simulink library "ddm"  (R2021b)
settings: Solver=VariableStepAuto  StartTime=0.0  StopTime=10.0  RelTol=1e-3
undefined symbols (not defined in the file or in its folder): ENUM_ADASACCSTA_ERROR, ENUM_ADASACCSTA_OFF, ENUM_ADASACCSTA_STANDBY, ENUM_ADASISASTA_OFF, ENUM_ALLOWMOV_ALLOWREADY, ENUM_APS, ENUM_BRKSTA_ERROR, ENUM_BRKSTA_OFF, ENUM_BRKSTA_ON, ENUM_CHGPREACTERRSTA_OBCPRE, ENUM_DCDCFAULTSTA_ANYFAULTLV1, ENUM_DCDCFAULTSTA_ANYFAULTLV2, ENUM_DRIVETRAIN_AWD, ENUM_DRIVETRAIN_FWD, ENUM_DRIVETRAIN_RWD, ENUM_DRSEATSTA_INVALID, ENUM_EDUDRTSTA_NORMAL, ENUM_EPBSTA_APPLIED, ENUM_EPBSTA_RELEASED, ENUM_HVBATTREADYPRE_READY, ENUM_MCUWARN_LV0, ENUM_MCUWARN_LV1, ENUM_MCUWARN_LV2, ENUM_MCUWARN_LV3, ENUM_MCUWARN_NOERROR, ENUM_OBCFAULTSTA_ANYFAULT, ENUM_PAS_R2F2, ENUM_PDFAULT_BATTPDFAIL, ENUM_PDFAULT_DCDCDISABLE, ENUM_PDFAULT_MCUDISABLE, ENUM_PDFAULT_MCUDISCHRG, ENUM_POWERSTA_OFF, ENUM_POWERSTA_ON, ENUM_POWERSTA_READY, ENUM_POWERSTA_STANDBY, ENUM_PRESSINDI_LOW, ENUM_PUFAULT_BATTUPFAIL, ENUM_PUFAULT_DCDCENABLEFAIL, ENUM_PUFAULT_PRECHRGCHKFAIL, ENUM_PUFAULT_SAFETYCHKFAIL, ENUM_PUSTATE_COMPLETED, ENUM_PWRSTASW_OFF, ENUM_PWRSTASW_OFFA, ENUM_PWRSTASW_OFFCHVCHRG, ENUM_PWRSTASW_OFFCLVCHRG, ENUM_PWRSTASW_ON, ENUM_PWRSTASW_ONHVCHRG, ENUM_PWRSTASW_READY, ENUM_PWRSTASW_STANDBY, ENUM_RANGESTA_12IN, ENUM_RANGESTA_12OUT, ENUM_SHIFTCOMMAND_D, ENUM_SHIFTCOMMAND_N, ENUM_SHIFTCOMMAND_P, ENUM_SHIFTCOMMAND_R, ENUM_ZONEMALFUNLV_1ST, ENUM_ZONEMALFUNLV_2ND, ENUM_ZONEMALFUNLV_3RD, ENUM_ZONEMALFUNLV_4TH, ENUM_ZONESPDCTRLMODE_ACC ... (+832)
libraries: hcu_lib x738, $bdroot x26, simulink x7
(part 16 of 25)

== system ddm/DDM/DDM/PMM/Fault level/Fault level 4 subsystem error ==
  note: Fail Safe Operation During Failure Detection
  note: Test Detection Criteria
  note: Diagnostics and Fault Handling
  note: Release Condition After Failure Decision
  note: Release Condition During Failure Detection
  note: Test Pass Criteria
  note: Fail Safe Operation After Failure Decision
  task_time_s : Inport
  VPMM_PowerSta_enum : Inport  Port=2
  VPMM_PwrStaSW_enum : Inport  Port=3
  VDDM_C3BMS6LCCFS_flg : Inport  Port=4
  VINP_BMSWarn7_flg : Inport  Port=5
  VINP_BMSWarn8_flg : Inport  Port=6
  DTC_clear_request : Inport  Port=7
  No_CAN3_BUS_OFF : Inport  Port=8
  Constant10 : Constant  Value=KDDM_Lv4ErrDetSW_flg
  Constant11 : Constant  Value=KDDM_Lv4ErrPassSW_flg
  Constant15 : Constant  Value=KDDM_Lv4ErrCFSSW_flg
  Constant16 : Constant  Value=TRUE
  Constant18 : Constant  Value=KDDM_Lv4ErrPassTO_s
  Constant19 : Constant  Value=ENUM_POWERSTA_OFF
  Constant{2,21,25,27} (4 alike) : Constant  Value=FALSE
  Constant20 : Constant  Value=KDDM_Lv4ErrDFSSW_flg
  Constant22 : Constant  Value=ENUM_PWRSTASW_OFF
  Constant23 : Constant  Value=TRUE
  Constant24 : Constant  Value=TRUE
  Constant26 : Constant  Value=ENUM_PWRSTASW_OFF
  Constant3 : Constant  Value=KDDM_Lv4ErrDetTO_s
  Constant4 : Constant  Value=KDDM_Lv4ErrPassTO_s
  Constant40 : Constant  Value=KDDM_Lv4ErrDTC_cnt
  Constant5 : Constant  Value=KDDM_Lv4ErrDTC_cnt
  DTC_Couter : hcu_lib/Basic_Blocks/DTC_Couter
  DTC_Info : hcu_lib/Basic_Blocks/DTC_Info
  Data Type Conversion1 : DataTypeConversion  OutDataTypeStr=uint8
  Equal : RelationalOperator  Operator=~=  OutDataTypeStr=boolean  RndMeth=Simplest
  Equal2 : RelationalOperator  Operator=~=  OutDataTypeStr=boolean  RndMeth=Simplest
  Equal3 : RelationalOperator  OutDataTypeStr=boolean  RndMeth=Simplest
  Equal4 : RelationalOperator  Operator===  OutDataTypeStr=boolean  RndMeth=Simplest
  Goto24 : Goto  Commented=on  GotoTag=VDDM_EDriveSysErrVCUErr_flg
  Logical Operator1 : Logic  Operator=NOT  AllPortsSameDT=off  OutDataTypeStr=boolean
  Logical Operator{3,5,8,11} (4 alike) : Logic  Operator=OR  AllPortsSameDT=off  OutDataTypeStr=boolean
  Logical Operator{12,15,18..19} (4 alike) : Logic  AllPortsSameDT=off  OutDataTypeStr=boolean
  Logical Operator2 : Logic  Inputs=3  AllPortsSameDT=off  OutDataTypeStr=boolean
  Logical Operator4 : Logic  Operator=NOT  AllPortsSameDT=off  OutDataTypeStr=boolean
  Logical Operator6 : Logic  Operator=NOT  AllPortsSameDT=off  OutDataTypeStr=boolean
  Logical Operator7 : Logic  Inputs=3  AllPortsSameDT=off  OutDataTypeStr=boolean
  Relay : Relay  OnSwitchValue=ONE_INT  OffSwitchValue=ZERO_INT
  SR_Latch1 : Subsystem  mask(SR_Latch){}
      mask help: SR latch function.
  SR_Latch3 : hcu_lib/Basic_Blocks/SR_Latch
  SR_Latch4 : hcu_lib/Basic_Blocks/SR_Latch
  Switch{,2,4..6} (5 alike) : Switch  Criteria=u2 ~= 0
  Test Detection Criteria : hcu_lib/Basic_Blocks/Test Detection Criteria
  Timer1 : hcu_lib/Basic_Blocks/Timer
  VDDM_Lv4ErrDTC_raw32 : Outport
  wires:
  VINP_BMSWarn8_flg/1 -> [VINP_BMSWarn8_flg]
  VPMM_PowerSta_enum/1 -> [VPMM_PowerSta_enum]
  VPMM_PwrStaSW_enum/1 -> [VPMM_PwrStaSW_enum]
  task_time_s/1 -> [task_time_s]
  VINP_BMSWarn7_flg/1 -> [VINP_BMSWarn7_flg]
  VDDM_C3BMS6LCCFS_flg/1 -> [VDDM_C3BMS6LCCFS_flg]
  [VDDM_Lv4ErrCFSRls_flg] -> Logical Operator3/2
  Constant10/1 -> Logical Operator19/2
  SR_Latch1/1(latched) -> [VDDM_Lv4ErrPass_flg]  "VDDM_Lv4ErrPass_flg"
  [VINP_BMSWarn7_flg] -> Logical Operator11/1
  Constant5/1 -> DTC_Couter/3
  Constant11/1 -> Logical Operator15/2
  Constant20/1 -> Logical Operator12/1
  [No_CAN3_BUS_OFF] -> Logical Operator2/1
  Logical Operator6/1 -> Timer1/1
  [task_time_s] -> Test Detection Criteria/2
  [VDDM_Lv4ErrCFS_flg] -> Switch/2
  [VDDM_C3BMS6LCCFS_flg] -> Logical Operator1/1
  DTC_Couter/2 -> Data Type Conversion1/1
  Switch/1 -> Goto24/1
  Equal3/1 -> SR_Latch1/1(set)
  Constant40/1 -> Test Detection Criteria/3
  Equal4/1 -> Logical Operator8/1
  [DTC_clear_request] -> Logical Operator8/2
  Timer1/1 -> Equal3/1
  Constant26/1 -> Equal/2
  Constant18/1 -> Equal3/2
  Logical Operator18/1 -> [VDDM_Lv4ErrCFS_flg]
  Data Type Conversion1/1 -> [VDDM_Lv4ErrDTC_cnt]  "VDDM_Lv4ErrDTC_cnt"
  Logical Operator1/1 -> Logical Operator2/3
  Constant24/1 -> Switch4/1
  SR_Latch3/1 -> Logical Operator12/2
  Logical Operator19/1 -> DTC_Couter/1
  Logical Operator15/1 -> DTC_Couter/2
  Logical Operator2/1 -> Switch5/2
  Logical Operator3/1 -> Logical Operator15/1
  Switch2/1 -> Logical Operator6/1, Timer1/2
  DTC_Couter/1 -> SR_Latch4/1
  Logical Operator8/1 -> Switch4/2
  Logical Operator12/1 -> [VDDM_Lv4ErrDFS_flg]
  Constant16/1 -> Switch/1
  Switch4/1 -> [VDDM_Lv4ErrCFSRls_flg]
  Constant15/1 -> Logical Operator18/2
  [VDDM_Lv4ErrCFSRls_flg] -> SR_Latch4/2
  [VDDM_Lv4ErrPass_flg] -> Logical Operator3/1
  Relay/1 -> SR_Latch3/1
  Constant27/1 -> Switch5/3
  Equal/1 -> Logical Operator2/2
  Constant21/1 -> Switch/3
  Test Detection Criteria/1 -> [VDDM_Lv4ErrDet_flg]  "VDDM_Lv4ErrDet_flg"
  Logical Operator11/1 -> Switch5/1
  Constant25/1 -> Switch4/3
  Constant19/1 -> Equal4/2
  [VDDM_Lv4ErrDTC_cnt] -> Relay/1
  Constant4/1 -> Timer1/4
  SR_Latch4/1 -> Logical Operator18/1
  [VDDM_Lv4ErrDet_flg] -> Logical Operator19/1
  [VINP_BMSWarn8_flg] -> Logical Operator11/2
  [VINP_BMSWarn8_flg] -> Logical Operator5/2
  Logical Operator5/1 -> Switch2/1
  Equal2/1 -> Logical Operator7/2
  Constant23/1 -> Switch2/3
  Constant22/1 -> Equal2/2
  Logical Operator7/1 -> Switch2/2
  Logical Operator4/1 -> Logical Operator7/3
  [VPMM_PwrStaSW_enum] -> Equal2/1
  [VDDM_C3BMS6LCCFS_flg] -> Logical Operator4/1
  [No_CAN3_BUS_OFF] -> Logical Operator7/1
  [VINP_BMSWarn7_flg] -> Logical Operator5/1
  [VPMM_PowerSta_enum] -> Equal4/1
  [VPMM_PwrStaSW_enum] -> Equal/1
  DTC_clear_request/1 -> [DTC_clear_request]
  No_CAN3_BUS_OFF/1 -> [No_CAN3_BUS_OFF]
  [task_time_s] -> Timer1/3
  DTC_Info/1 -> VDDM_Lv4ErrDTC_raw32/1  "VDDM_Lv4ErrDTC_raw32"
  [VDDM_Lv4ErrPass_flg] -> DTC_Info/2
  [VDDM_Lv4ErrCFS_flg] -> DTC_Info/3
  [VDDM_Lv4ErrCFS_flg] -> SR_Latch3/2
  [VDDM_Lv4ErrDet_flg] -> DTC_Info/1
  Constant3/1 -> Test Detection Criteria/4
  [DTC_clear_request] -> DTC_Info/4
  [DTC_clear_request] -> Switch6/2
  Switch6/1 -> Test Detection Criteria/1
  Switch5/1 -> [VDDM_xxx_flg], Switch6/3
  Constant2/1 -> Switch6/1
  [VDDM_xxx_flg] -> SR_Latch1/2(reset)

== system ddm/DDM/DDM/PMM/Key authentication failed/SR_Latch1 ==
  set : Inport
  reset : Inport  Port=2
  Logical Operator : Logic  AllPortsSameDT=off  OutDataTypeStr=boolean
  Logical Operator1 : Logic  Operator=NOT  AllPortsSameDT=off  OutDataTypeStr=boolean
  Switch1 : Switch  Criteria=u2 ~= 0  Threshold=0.5
      settings: AttributesFormatString=<Criteria=%<Criteria>>
  Switch2 : Switch  Criteria=u2 ~= 0  Threshold=0.5
      settings: AttributesFormatString=<Criteria=%<Criteria>>
  Unit Delay : UnitDelay  SampleTime=-1  HasFrameUpgradeWarning=on
  latched : Outport
  wires:
  Switch1/1 -> Unit Delay/1, latched/1
  set/1 -> Switch1/1, Logical Operator/1
  reset/1 -> Switch2/2, Logical Operator1/1
  Unit Delay/1 -> Switch2/3
  Switch2/1 -> Switch1/3
  Logical Operator/1 -> Switch1/2
  Logical Operator1/1 -> Logical Operator/2, Switch2/1

== system ddm/DDM/DDM/PMM/LV/Initial LV battery voltage too low ==
  note: Test Detection Criteria
  note: Test Pass Criteria
  note: Fail Safe After Decision
  note: Fail Safe During Detection
  note: Release Condition During Detection
  note: Release Condition After Decision
  note: Diagnostics and Fault Handling
  task_time_s : Inport
  VPMM_PowerSta_enum : Inport  Port=2
  VPMM_PwrStaSW_enum : Inport  Port=3
  VINP_LVBattDet12V_V : Inport  Port=4
  VINP_CANMsgValidBMS2_flg : Inport  Port=5
  DTC_clear_request : Inport  Port=6
  Constant1 : Constant  Value=TRUE
  Constant10 : Constant  Value=ENUM_POWERSTA_OFF
  Constant11 : Constant  Value=KDDM_IniLVLoPassSW_flg
  Constant15 : Constant  Value=KDDM_IniLVLoCFSSW_flg
  Constant16 : Constant  Value=TRUE
  Constant18 : Constant  Value=KDDM_IniLVLoPassTO_s
  Constant19 : Constant  Value=KDDM_IniLVLoPassTO_s
  Constant2 : Constant  Value=ENUM_PWRSTASW_STANDBY
  Constant20 : Constant  Value=KDDM_IniLVLoDFSSW_flg
  Constant{4,8,21,25} (4 alike) : Constant  Value=FALSE
  Constant24 : Constant  Value=TRUE
  Constant3 : Constant  Value=ENUM_PWRSTASW_OFF
  Constant40 : Constant  Value=KDDM_IniLVLoDTC_cnt
  Constant41 : Constant  Value=KDDM_IniLVLoDetTO_s
  Constant46 : Constant  Value=KDDM_IniLVLoDetSW_flg
  Constant48 : Constant  Value=KDDM_IniLVLoDTC_cnt
  Constant5 : Constant  Value=ENUM_PWRSTASW_STANDBY
  Constant6 : Constant  Value=KDDM_IniLVLoThd_mv
  Constant7 : Constant  Value=ENUM_PWRSTASW_OFF
  Constant9 : Constant  Value=KDDM_IniLVLoThd_mv
  DTC_Couter : hcu_lib/Basic_Blocks/DTC_Couter
  DTC_Info : hcu_lib/Basic_Blocks/DTC_Info
  Data Type Conversion1 : DataTypeConversion  OutDataTypeStr=uint8
  Equal{,1..2,4,6} (5 alike) : RelationalOperator  Operator===  OutDataTypeStr=boolean  RndMeth=Simplest
  Equal3 : RelationalOperator  OutDataTypeStr=boolean  RndMeth=Simplest
  Equal5 : RelationalOperator  Operator=<=  OutDataTypeStr=boolean  RndMeth=Simplest
  Equal7 : RelationalOperator  Operator=<=  OutDataTypeStr=boolean  RndMeth=Simplest
  Gain1 : Gain  Gain=1000
  Gain2 : Gain  Gain=1000
  Goto6 : Goto  Commented=on  GotoTag=VDDM_EDriveSysErrVCUErr_flg
  Logical Operator{1..2,12,15,18..19} (6 alike) : Logic  AllPortsSameDT=off  OutDataTypeStr=boolean
  Logical Operator3 : Logic  Operator=OR  AllPortsSameDT=off  OutDataTypeStr=boolean
  Logical Operator6 : Logic  Operator=NOT  AllPortsSameDT=off  OutDataTypeStr=boolean
  Logical Operator8 : Logic  Operator=OR  AllPortsSameDT=off  OutDataTypeStr=boolean
  OR : Logic  Operator=OR  AllPortsSameDT=off  OutDataTypeStr=boolean
  OR1 : Logic  Operator=OR  AllPortsSameDT=off  OutDataTypeStr=boolean
  Relay : Relay  OnSwitchValue=ONE_INT  OffSwitchValue=ZERO_INT
  SR_Latch1 : Subsystem  mask(SR_Latch){}
      mask help: SR latch function.
  SR_Latch3 : hcu_lib/Basic_Blocks/SR_Latch
  SR_Latch4 : hcu_lib/Basic_Blocks/SR_Latch
  Switch{,2..4,6} (5 alike) : Switch  Criteria=u2 ~= 0
  Test Detection Criteria : hcu_lib/Basic_Blocks/Test Detection Criteria
  Timer1 : hcu_lib/Basic_Blocks/Timer
  VDDM_IniLVLoDTC_raw32 : Outport
  wires:
  task_time_s/1 -> [task_time_s]
  VINP_LVBattDet12V_V/1 -> [VINP_LVBattDet12V_V]
  VPMM_PwrStaSW_enum/1 -> [VPMM_PwrStaSW_enum]
  VPMM_PowerSta_enum/1 -> [VPMM_PowerSta_enum]
  Logical Operator2/1 -> Switch3/2
  [task_time_s] -> Test Detection Criteria/2
  Test Detection Criteria/1 -> [VDDM_IniLVLoDet_flg]  "VDDM_IniLVLoDet_flg"
  Constant40/1 -> Test Detection Criteria/3
  Constant3/1 -> Equal/2
  Constant4/1 -> Switch3/3
  [VPMM_PwrStaSW_enum] -> Equal1/2, Equal/1
  SR_Latch1/1(latched) -> [VDDM_IniLVLoPass_flg]  "VDDM_IniLVLoPass_flg"
  Equal3/1 -> SR_Latch1/1(set)
  Logical Operator6/1 -> Timer1/1
  Constant19/1 -> Equal3/2
  Switch4/1 -> Logical Operator6/1, Timer1/2
  Timer1/1 -> Equal3/1
  Constant18/1 -> Timer1/4
  Constant16/1 -> Switch4/3
  [VDDM_IniLVLoCFS_flg] -> Switch/2
  Switch/1 -> Goto6/1
  Constant1/1 -> Switch/1
  Constant21/1 -> Switch/3
  Logical Operator8/1 -> Switch2/2
  Constant25/1 -> Switch2/3
  Switch2/1 -> [VDDM_IniLVLoCFSRls_flg]
  [DTC_clear_request] -> Logical Operator8/2
  Constant24/1 -> Switch2/1
  Constant10/1 -> Equal4/2
  Equal4/1 -> Logical Operator8/1
  [VDDM_IniLVLoDTC_cnt] -> Relay/1
  Logical Operator3/1 -> Logical Operator15/1
  [VDDM_IniLVLoDet_flg] -> Logical Operator19/1
  Relay/1 -> SR_Latch3/1
  DTC_Couter/2 -> Data Type Conversion1/1
  Constant48/1 -> DTC_Couter/3
  Logical Operator15/1 -> DTC_Couter/2
  Constant11/1 -> Logical Operator15/2
  Logical Operator19/1 -> DTC_Couter/1
  Constant46/1 -> Logical Operator19/2
  Data Type Conversion1/1 -> [VDDM_IniLVLoDTC_cnt]  "VDDM_IniLVLoDTC_cnt"
  DTC_Couter/1 -> SR_Latch4/1
  [VDDM_IniLVLoPass_flg] -> Logical Operator3/1
  [VDDM_IniLVLoCFSRls_flg] -> SR_Latch4/2
  SR_Latch4/1 -> Logical Operator18/1
  Logical Operator12/1 -> [VDDM_IniLVLoDFS_flg]
  Constant15/1 -> Logical Operator18/2
  SR_Latch3/1 -> Logical Operator12/2
  Constant20/1 -> Logical Operator12/1
  Logical Operator18/1 -> [VDDM_IniLVLoCFS_flg]
  [VDDM_IniLVLoCFSRls_flg] -> Logical Operator3/2
  DTC_clear_request/1 -> [DTC_clear_request]
  VINP_CANMsgValidBMS2_flg/1 -> [VINP_CANMsgValidBMS2_flg]
  [VINP_CANMsgValidBMS2_flg] -> Logical Operator2/2
  Equal/1 -> OR/2
  OR/1 -> Logical Operator2/1
  Equal1/1 -> OR/1
  Constant2/1 -> Equal1/1
  [VINP_LVBattDet12V_V] -> Gain1/1
  Equal5/1 -> Switch3/1
  Constant6/1 -> Equal5/2
  Gain1/1 -> Equal5/1
  Equal7/1 -> Switch4/1
  [VINP_CANMsgValidBMS2_flg] -> Logical Operator1/2
  [VPMM_PwrStaSW_enum] -> Equal6/2, Equal2/1
  Equal6/1 -> OR1/1
  Logical Operator1/1 -> Switch4/2
  Constant7/1 -> Equal2/2
  Gain2/1 -> Equal7/1
  [VINP_LVBattDet12V_V] -> Gain2/1
  Constant9/1 -> Equal7/2
  OR1/1 -> Logical Operator1/1
  Equal2/1 -> OR1/2
  Constant5/1 -> Equal6/1
  [task_time_s] -> Timer1/3
  [VPMM_PowerSta_enum] -> Equal4/1
  DTC_Info/1 -> VDDM_IniLVLoDTC_raw32/1  "VDDM_IniLVLoDTC_raw32"
  [VDDM_IniLVLoPass_flg] -> DTC_Info/2
  [VDDM_IniLVLoCFS_flg] -> DTC_Info/3
  [VDDM_IniLVLoCFS_flg] -> SR_Latch3/2
  [VDDM_IniLVLoDet_flg] -> DTC_Info/1
  Constant41/1 -> Test Detection Criteria/4
  [DTC_clear_request] -> DTC_Info/4
  [DTC_clear_request] -> Switch6/2
  Switch6/1 -> Test Detection Criteria/1
  Switch3/1 -> [VDDM_xxx_flg], Switch6/3
  Constant8/1 -> Switch6/1
  [VDDM_xxx_flg] -> SR_Latch1/2(reset)

== system ddm/DDM/DDM/PMM/LV/LV power supply voltage too high ==
  note: Release Condition During Detection
  note: Fail Safe During Detection
  note: Diagnostics and Fault Handling
  note: Test Detection Criteria
  note: Fail Safe After Decision
  note: Test Pass Criteria
  note: Release Condition After Decision
  task_time_s : Inport
  VPMM_PowerSta_enum : Inport  Port=2
  VPMM_PwrStaSW_enum : Inport  Port=3
  VINP_LVBattDet12V_V : Inport  Port=4
  VINP_CANMsgValidBMS2_flg : Inport  Port=5
  DTC_clear_request : Inport  Port=6
  Constant1 : Constant  Value=TRUE
  Constant10 : Constant  Value=ENUM_POWERSTA_OFF
  Constant11 : Constant  Value=KDDM_LVSupHiPassSW_flg
  Constant12 : Constant  Value=ENUM_PWRSTASW_READY
  Constant13 : Constant  Value=ENUM_PWRSTASW_ON
  Constant14 : Constant  Value=ENUM_PWRSTASW_OFFCLVCHRG
  Constant15 : Constant  Value=KDDM_LVSupHiCFSSW_flg
  Constant16 : Constant  Value=TRUE
  Constant17 : Constant  Value=ENUM_PWRSTASW_OFFCHVCHRG
  Constant18 : Constant  Value=KDDM_LVSupHiPassTO_s
  Constant19 : Constant  Value=KDDM_LVSupHiPassTO_s
  Constant2 : Constant  Value=ENUM_PWRSTASW_ON
  Constant20 : Constant  Value=KDDM_LVSupHiDFSSW_flg
  Constant{4,21,25,27} (4 alike) : Constant  Value=FALSE
  Constant22 : Constant  Value=ENUM_PWRSTASW_OFFCLVCHRG
  Constant23 : Constant  Value=ENUM_PWRSTASW_ONHVCHRG
  Constant24 : Constant  Value=TRUE
  Constant26 : Constant  Value=ENUM_PWRSTASW_OFFA
  Constant3 : Constant  Value=ENUM_PWRSTASW_ONHVCHRG
  Constant40 : Constant  Value=KDDM_LVSupHiDTC_cnt
  Constant41 : Constant  Value=KDDM_LVSupHiDetTO_s
  Constant46 : Constant  Value=KDDM_LVSupHiDetSW_flg
  Constant48 : Constant  Value=KDDM_LVSupHiDTC_cnt
  Constant5 : Constant  Value=ENUM_PWRSTASW_READY
  Constant6 : Constant  Value=KDDM_LVSupHiThd_mv
  Constant7 : Constant  Value=ENUM_PWRSTASW_OFFCHVCHRG
  Constant8 : Constant  Value=ENUM_PWRSTASW_OFFA
  Constant9 : Constant  Value=KDDM_LVSupHiThd_mv
  DTC_Couter : hcu_lib/Basic_Blocks/DTC_Couter
  DTC_Info : hcu_lib/Basic_Blocks/DTC_Info
  Data Type Conversion1 : DataTypeConversion  OutDataTypeStr=uint8
  Equal{,1..2,4,6,8..15} (13 alike) : RelationalOperator  Operator===  OutDataTypeStr=boolean  RndMeth=Simplest
  Equal3 : RelationalOperator  OutDataTypeStr=boolean  RndMeth=Simplest
  Equal5 : RelationalOperator  OutDataTypeStr=boolean  RndMeth=Simplest
  Equal7 : RelationalOperator  OutDataTypeStr=boolean  RndMeth=Simplest
  Gain1 : Gain  Gain=KXX2XX
  Gain2 : Gain  Gain=KXX2XX
  Goto6 : Goto  Commented=on  GotoTag=VDDM_EDriveSysErrVCUErr_flg
  Logical Operator{1..2,12,15,18..19} (6 alike) : Logic  AllPortsSameDT=off  OutDataTypeStr=boolean
  Logical Operator3 : Logic  Operator=OR  AllPortsSameDT=off  OutDataTypeStr=boolean
  Logical Operator6 : Logic  Operator=NOT  AllPortsSameDT=off  OutDataTypeStr=boolean
  Logical Operator8 : Logic  Operator=OR  AllPortsSameDT=off  OutDataTypeStr=boolean
  OR : Logic  Operator=OR  Inputs=6  AllPortsSameDT=off  OutDataTypeStr=boolean
  OR1 : Logic  Operator=OR  Inputs=6  AllPortsSameDT=off  OutDataTypeStr=boolean
  Relay : Relay  OnSwitchValue=ONE_INT  OffSwitchValue=ZERO_INT
  SR_Latch1 : Subsystem  mask(SR_Latch){}
      mask help: SR latch function.
  SR_Latch3 : hcu_lib/Basic_Blocks/SR_Latch
  SR_Latch4 : hcu_lib/Basic_Blocks/SR_Latch
  Switch{,2..4,6} (5 alike) : Switch  Criteria=u2 ~= 0
  Test Detection Criteria : hcu_lib/Basic_Blocks/Test Detection Criteria
  Timer1 : hcu_lib/Basic_Blocks/Timer
  VDDM_LVSupHiDTC_raw32 : Outport
  wires:
  task_time_s/1 -> [task_time_s]
  VINP_LVBattDet12V_V/1 -> [VINP_LVBattDet12V_V]
  DTC_clear_request/1 -> [DTC_clear_request]
  VINP_CANMsgValidBMS2_flg/1 -> [VINP_CANMsgValidBMS2_flg]
  Equal3/1 -> SR_Latch1/1(set)
  SR_Latch1/1(latched) -> [VDDM_LVSupHiPass_flg]
  Constant4/1 -> Switch3/3
  Test Detection Criteria/1 -> [VDDM_LVSupHiDet_flg]  "VDDM_LVSupHiDet_flg"
  Logical Operator3/1 -> Logical Operator15/1
  Logical Operator19/1 -> DTC_Couter/1
  Constant20/1 -> Logical Operator12/1
  [task_time_s] -> Test Detection Criteria/2
  Constant11/1 -> Logical Operator15/2
  Timer1/1 -> Equal3/1
  SR_Latch3/1 -> Logical Operator12/2
  Logical Operator15/1 -> DTC_Couter/2
  Logical Operator12/1 -> [VDDM_LVSupHiDFS_flg]
  Data Type Conversion1/1 -> [VDDM_LVSupHiDTC_cnt]  "VDDM_LVSupHiDTC_cnt"
  [VDDM_LVSupHiCFSRls_flg] -> Logical Operator3/2
  Relay/1 -> SR_Latch3/1
  [VDDM_LVSupHiPass_flg] -> Logical Operator3/1
  DTC_Couter/1 -> SR_Latch4/1
  SR_Latch4/1 -> Logical Operator18/1
  Switch/1 -> Goto6/1
  [VDDM_LVSupHiDet_flg] -> Logical Operator19/1
  [VDDM_LVSupHiDTC_cnt] -> Relay/1
  Equal4/1 -> Logical Operator8/1
  [VDDM_LVSupHiCFS_flg] -> Switch/2
  Constant21/1 -> Switch/3
  Constant10/1 -> Equal4/2
  Constant24/1 -> Switch2/1
  Logical Operator8/1 -> Switch2/2
  Switch4/1 -> Logical Operator6/1, Timer1/2
  Constant1/1 -> Switch/1
  Constant40/1 -> Test Detection Criteria/3
  Constant9/1 -> Equal7/2
  Gain2/1 -> Equal7/1
  [VINP_LVBattDet12V_V] -> Gain2/1
  Constant18/1 -> Timer1/4
  Constant48/1 -> DTC_Couter/3
  [VINP_LVBattDet12V_V] -> Gain1/1
  Switch2/1 -> [VDDM_LVSupHiCFSRls_flg]
  [VDDM_LVSupHiCFSRls_flg] -> SR_Latch4/2
  DTC_Couter/2 -> Data Type Conversion1/1
  Gain1/1 -> Equal5/1
  Equal7/1 -> Switch4/1
  Constant15/1 -> Logical Operator18/2
  [DTC_clear_request] -> Logical Operator8/2
  Logical Operator18/1 -> [VDDM_LVSupHiCFS_flg]
  Constant16/1 -> Switch4/3
  Constant46/1 -> Logical Operator19/2
  Constant25/1 -> Switch2/3
  Equal5/1 -> Switch3/1
  [VPMM_PowerSta_enum] -> Equal4/1
  Logical Operator6/1 -> Timer1/1
  Constant19/1 -> Equal3/2
  Constant6/1 -> Equal5/2
  [task_time_s] -> Timer1/3
  VPMM_PowerSta_enum/1 -> [VPMM_PowerSta_enum]
  VPMM_PwrStaSW_enum/1 -> [VPMM_PwrStaSW_enum]
  DTC_Info/1 -> VDDM_LVSupHiDTC_raw32/1  "VDDM_LVSupHiDTC_raw32"
  [VDDM_LVSupHiPass_flg] -> DTC_Info/2
  [VDDM_LVSupHiCFS_flg] -> DTC_Info/3
  [VDDM_LVSupHiCFS_flg] -> SR_Latch3/2
  [VDDM_LVSupHiDet_flg] -> DTC_Info/1
  Constant41/1 -> Test Detection Criteria/4
  Equal12/1 -> OR/5
  Constant22/1 -> Equal13/2
  [VPMM_PwrStaSW_enum] -> Equal12/2, Equal13/1
  Equal13/1 -> OR/6
  Constant3/1 -> Equal/2
  Constant8/1 -> Equal8/2
  Equal/1 -> OR/2
  [VINP_CANMsgValidBMS2_flg] -> Logical Operator2/2
  Equal1/1 -> OR/1
  OR/1 -> Logical Operator2/1
  [VPMM_PwrStaSW_enum] -> Equal9/2, Equal8/1
  Constant12/1 -> Equal9/1
  Equal9/1 -> OR/3
  Logical Operator2/1 -> Switch3/2
  Constant2/1 -> Equal1/1
  [VPMM_PwrStaSW_enum] -> Equal1/2, Equal/1
  Equal8/1 -> OR/4
  Constant17/1 -> Equal12/1
  Equal10/1 -> OR1/5
  Constant14/1 -> Equal11/2
  [VPMM_PwrStaSW_enum] -> Equal10/2, Equal11/1
  Equal11/1 -> OR1/6
  Constant23/1 -> Equal2/2
  Constant26/1 -> Equal14/2
  Equal2/1 -> OR1/2
  [VINP_CANMsgValidBMS2_flg] -> Logical Operator1/2
  Equal6/1 -> OR1/1
  OR1/1 -> Logical Operator1/1
  [VPMM_PwrStaSW_enum] -> Equal15/2, Equal14/1
  Constant5/1 -> Equal15/1
  Equal15/1 -> OR1/3
  Logical Operator1/1 -> Switch4/2
  Constant13/1 -> Equal6/1
  [VPMM_PwrStaSW_enum] -> Equal6/2, Equal2/1
  Equal14/1 -> OR1/4
  Constant7/1 -> Equal10/1
  [DTC_clear_request] -> DTC_Info/4
  [DTC_clear_request] -> Switch6/2
  Switch6/1 -> Test Detection Criteria/1
  Switch3/1 -> [VDDM_xxx_flg], Switch6/3
  Constant27/1 -> Switch6/1
  [VDDM_xxx_flg] -> SR_Latch1/2(reset)

== system ddm/DDM/DDM/PMM/LV/LV power supply voltage too low ==
  note: Test Detection Criteria
  note: Test Pass Criteria
  note: Fail Safe After Decision
  note: Fail Safe During Detection
  note: Release Condition During Detection
  note: Release Condition After Decision
  note: Diagnostics and Fault Handling
  task_time_s : Inport
  VPMM_PowerSta_enum : Inport  Port=2
  VPMM_PwrStaSW_enum : Inport  Port=3
  VINP_LVBattDet12V_V : Inport  Port=4
  VINP_CANMsgValidBMS2_flg : Inport  Port=5
  DTC_clear_request : Inport  Port=6
  Constant1 : Constant  Value=TRUE
  Constant10 : Constant  Value=ENUM_POWERSTA_OFF
  Constant11 : Constant  Value=KDDM_LVSupLoPassSW_flg
  Constant12 : Constant  Value=ENUM_PWRSTASW_READY
  Constant13 : Constant  Value=ENUM_PWRSTASW_ON
  Constant14 : Constant  Value=ENUM_PWRSTASW_OFFCLVCHRG
  Constant15 : Constant  Value=KDDM_LVSupLoCFSSW_flg
  Constant16 : Constant  Value=TRUE
  Constant17 : Constant  Value=ENUM_PWRSTASW_OFFCHVCHRG
  Constant18 : Constant  Value=KDDM_LVSupLoPassTO_s
  Constant19 : Constant  Value=KDDM_LVSupLoPassTO_s
  Constant2 : Constant  Value=ENUM_PWRSTASW_ON
  Constant20 : Constant  Value=KDDM_LVSupLoDFSSW_flg
  Constant{4,21,25,27} (4 alike) : Constant  Value=FALSE
  Constant22 : Constant  Value=ENUM_PWRSTASW_OFFCLVCHRG
  Constant23 : Constant  Value=ENUM_PWRSTASW_ONHVCHRG
  Constant24 : Constant  Value=TRUE
  Constant26 : Constant  Value=ENUM_PWRSTASW_OFFA
  Constant3 : Constant  Value=ENUM_PWRSTASW_ONHVCHRG
  Constant40 : Constant  Value=KDDM_LVSupLoDTC_cnt
  Constant41 : Constant  Value=KDDM_LVSupLoDetTO_s
  Constant46 : Constant  Value=KDDM_LVSupLoDetSW_flg
  Constant48 : Constant  Value=KDDM_LVSupLoDTC_cnt
  Constant5 : Constant  Value=ENUM_PWRSTASW_READY
  Constant6 : Constant  Value=KDDM_LVSupLoThd_mv
  Constant7 : Constant  Value=ENUM_PWRSTASW_OFFCHVCHRG
  Constant8 : Constant  Value=ENUM_PWRSTASW_OFFA
  Constant9 : Constant  Value=KDDM_LVSupLoThd_mv
  DTC_Couter : hcu_lib/Basic_Blocks/DTC_Couter
  DTC_Info : hcu_lib/Basic_Blocks/DTC_Info
  Data Type Conversion1 : DataTypeConversion  OutDataTypeStr=uint8
  Equal{,1..2,4,6,8..15} (13 alike) : RelationalOperator  Operator===  OutDataTypeStr=boolean  RndMeth=Simplest
  Equal3 : RelationalOperator  OutDataTypeStr=boolean  RndMeth=Simplest
  Equal5 : RelationalOperator  Operator=<=  OutDataTypeStr=boolean  RndMeth=Simplest
  Equal7 : RelationalOperator  Operator=<=  OutDataTypeStr=boolean  RndMeth=Simplest
  Gain1 : Gain  Gain=1000
  Gain2 : Gain  Gain=1000
  Goto6 : Goto  Commented=on  GotoTag=VDDM_EDriveSysErrVCUErr_flg
  Logical Operator{1..2,12,15,18..19} (6 alike) : Logic  AllPortsSameDT=off  OutDataTypeStr=boolean
  Logical Operator3 : Logic  Operator=OR  AllPortsSameDT=off  OutDataTypeStr=boolean
  Logical Operator6 : Logic  Operator=NOT  AllPortsSameDT=off  OutDataTypeStr=boolean
  Logical Operator8 : Logic  Operator=OR  AllPortsSameDT=off  OutDataTypeStr=boolean
  OR : Logic  Operator=OR  Inputs=6  AllPortsSameDT=off  OutDataTypeStr=boolean
  OR1 : Logic  Operator=OR  Inputs=6  AllPortsSameDT=off  OutDataTypeStr=boolean
  Relay : Relay  OnSwitchValue=ONE_INT  OffSwitchValue=ZERO_INT
  SR_Latch1 : Subsystem  mask(SR_Latch){}
      mask help: SR latch function.
  SR_Latch3 : hcu_lib/Basic_Blocks/SR_Latch
  SR_Latch4 : hcu_lib/Basic_Blocks/SR_Latch
  Switch{,2..4,6} (5 alike) : Switch  Criteria=u2 ~= 0
  Test Detection Criteria : hcu_lib/Basic_Blocks/Test Detection Criteria
  Timer1 : hcu_lib/Basic_Blocks/Timer
  VDDM_LVSupLoDTC_raw32 : Outport
  wires:
  task_time_s/1 -> [task_time_s]
  VINP_LVBattDet12V_V/1 -> [VINP_LVBattDet12V_V]
  VPMM_PwrStaSW_enum/1 -> [VPMM_PwrStaSW_enum]
  VPMM_PowerSta_enum/1 -> [VPMM_PowerSta_enum]
  Logical Operator2/1 -> Switch3/2
  [task_time_s] -> Test Detection Criteria/2
  Test Detection Criteria/1 -> [VDDM_LVSupLoDet_flg]  "VDDM_LVSupLoDet_flg"
  Constant40/1 -> Test Detection Criteria/3
  Constant3/1 -> Equal/2
  Constant4/1 -> Switch3/3
  [VPMM_PwrStaSW_enum] -> Equal1/2, Equal/1
  SR_Latch1/1(latched) -> [VDDM_LVSupLoPass_flg]
  Equal3/1 -> SR_Latch1/1(set)
  Logical Operator6/1 -> Timer1/1
  Constant19/1 -> Equal3/2
  Switch4/1 -> Logical Operator6/1, Timer1/2
  Timer1/1 -> Equal3/1
  Constant18/1 -> Timer1/4
  Constant16/1 -> Switch4/3
  [VDDM_LVSupLoCFS_flg] -> Switch/2
  Switch/1 -> Goto6/1
  Constant1/1 -> Switch/1
  Constant21/1 -> Switch/3
  Logical Operator8/1 -> Switch2/2
  Constant25/1 -> Switch2/3
  Switch2/1 -> [VDDM_LVSupLoCFSRls_flg]
  [DTC_clear_request] -> Logical Operator8/2
  Constant24/1 -> Switch2/1
  Constant10/1 -> Equal4/2
  Equal4/1 -> Logical Operator8/1
  [VDDM_LVSupLoDTC_cnt] -> Relay/1
  Logical Operator3/1 -> Logical Operator15/1
  [VDDM_LVSupLoDet_flg] -> Logical Operator19/1
  Relay/1 -> SR_Latch3/1
  DTC_Couter/2 -> Data Type Conversion1/1
  Constant48/1 -> DTC_Couter/3
  Logical Operator15/1 -> DTC_Couter/2
  Constant11/1 -> Logical Operator15/2
  Logical Operator19/1 -> DTC_Couter/1
  Constant46/1 -> Logical Operator19/2
  Data Type Conversion1/1 -> [VDDM_LVSupLoDTC_cnt]  "VDDM_LVSupLoDTC_cnt"
  DTC_Couter/1 -> SR_Latch4/1
  [VDDM_LVSupLoPass_flg] -> Logical Operator3/1
  [VDDM_LVSupLoCFSRls_flg] -> SR_Latch4/2
  SR_Latch4/1 -> Logical Operator18/1
  Logical Operator12/1 -> [VDDM_LVSupLoDFS_flg]
  Constant15/1 -> Logical Operator18/2
  SR_Latch3/1 -> Logical Operator12/2
  Constant20/1 -> Logical Operator12/1
  Logical Operator18/1 -> [VDDM_LVSupLoCFS_flg]
  [VDDM_LVSupLoCFSRls_flg] -> Logical Operator3/2
  DTC_clear_request/1 -> [DTC_clear_request]
  VINP_CANMsgValidBMS2_flg/1 -> [VINP_CANMsgValidBMS2_flg]
  [VINP_CANMsgValidBMS2_flg] -> Logical Operator2/2
  Equal/1 -> OR/2
  OR/1 -> Logical Operator2/1
  Equal1/1 -> OR/1
  Constant2/1 -> Equal1/1
  [VINP_LVBattDet12V_V] -> Gain1/1
  Equal5/1 -> Switch3/1
  Constant6/1 -> Equal5/2
  Gain1/1 -> Equal5/1
  Equal7/1 -> Switch4/1
  Gain2/1 -> Equal7/1
  [VINP_LVBattDet12V_V] -> Gain2/1
  Constant9/1 -> Equal7/2
  Constant8/1 -> Equal8/2
  [VPMM_PwrStaSW_enum] -> Equal9/2, Equal8/1
  Constant12/1 -> Equal9/1
  Equal9/1 -> OR/3
  Equal8/1 -> OR/4
  [task_time_s] -> Timer1/3
  [VPMM_PowerSta_enum] -> Equal4/1
  DTC_Info/1 -> VDDM_LVSupLoDTC_raw32/1  "VDDM_LVSupLoDTC_raw32"
  [VDDM_LVSupLoPass_flg] -> DTC_Info/2
  [VDDM_LVSupLoCFS_flg] -> DTC_Info/3
  [VDDM_LVSupLoCFS_flg] -> SR_Latch3/2
  [VDDM_LVSupLoDet_flg] -> DTC_Info/1
  Constant41/1 -> Test Detection Criteria/4
  [VPMM_PwrStaSW_enum] -> Equal12/2, Equal13/1
  Constant17/1 -> Equal12/1
  Constant22/1 -> Equal13/2
  Equal12/1 -> OR/5
  Equal13/1 -> OR/6
  Equal10/1 -> OR1/5
  Constant14/1 -> Equal11/2
  [VPMM_PwrStaSW_enum] -> Equal10/2, Equal11/1
  Equal11/1 -> OR1/6
  Constant23/1 -> Equal2/2
  Constant26/1 -> Equal14/2
  Equal2/1 -> OR1/2
  [VINP_CANMsgValidBMS2_flg] -> Logical Operator1/2
  Equal6/1 -> OR1/1
  OR1/1 -> Logical Operator1/1
  [VPMM_PwrStaSW_enum] -> Equal15/2, Equal14/1
  Constant5/1 -> Equal15/1
  Equal15/1 -> OR1/3
  Logical Operator1/1 -> Switch4/2
  Constant13/1 -> Equal6/1
  [VPMM_PwrStaSW_enum] -> Equal6/2, Equal2/1
  Equal14/1 -> OR1/4
  Constant7/1 -> Equal10/1
  [DTC_clear_request] -> DTC_Info/4
  [DTC_clear_request] -> Switch6/2
  Switch6/1 -> Test Detection Criteria/1
  Switch3/1 -> [VDDM_xxx_flg], Switch6/3
  Constant27/1 -> Switch6/1
  [VDDM_xxx_flg] -> SR_Latch1/2(reset)

== system ddm/DDM/DDM/PMM/SW failure/Driver seat switch failure ==
  note: Fail Safe During Detection
  note: Fail Safe After Decision
  note: Release Condition After Decision
  note: Release Condition During Detection
  note: Diagnostics and Fault Handling
  note: Test Pass Criteria
  note: Test Detection Criteria
  task_time_s : Inport
  VPMM_PowerSta_enum : Inport  Port=2
  VPMM_PwrStaSW_enum : Inport  Port=3
  VINP_DrStSW : Inport  Port=4
  DTC_clear_request : Inport  Port=5
  Add2 : Sum
  Add3 : Sum
  Add4 : Sum  AccumDataTypeStr=uint16
  Constant{1..2,12..13,31} (5 alike) : Constant  Value=ZERO_INT
  Constant10 : Constant  Value=KDDM_DrStSWDetTO_s
  Constant11 : Constant  Value=KDDM_DrStSWDTC_cnt
  Constant14 : Constant  Value=KDDM_DrStSW_s
  Constant28 : Constant  Value=ZERO_FLOAT
  Constant29 : Constant  Value=ONE_INT
  Constant3 : Constant  Value=ONE_INT
  Constant37 : Constant  Value=ENUM_PWRSTASW_OFF
  Constant39 : Constant  Value=KDDM_DrStSWPassTO_s
  Constant4 : Constant  Value=KDDM_DrStSW_s
  Constant42 : Constant  Value=ENUM_DRSEATSTA_INVALID
  Constant45 : Constant  Value=ENUM_POWERSTA_OFF
  Constant47 : Constant  Value=TRUE
  Constant49 : Constant  Value=KDDM_DrStSW_s
  Constant5 : Constant  Value=KDDM_DrStSWPassTO_s
  Constant50 : Constant  Value=ENUM_PWRSTASW_OFF
  Constant52 : Constant  Value=TRUE
  Constant53 : Constant  Value=FALSE
  Constant54 : Constant  Value=TRUE
  Constant55 : Constant  Value=FALSE
  Constant56 : Constant  Value=KDDM_DrStSWPassSW_flg
  Constant57 : Constant  Value=KDDM_DrStSWCFSSW_flg
  Constant58 : Constant  Value=KDDM_DrStSWDFSSW_flg
  Constant59 : Constant  Value=KDDM_DrStSWDetSW_flg
  Constant6 : Constant  Value=KDDM_DrStSWDetTO_s
  Constant60 : Constant  Value=KDDM_DrStSWDTC_cnt
  Constant7 : Constant  Value=FALSE
  DTC_Couter1 : hcu_lib/Basic_Blocks/DTC_Couter
  DTC_Info : hcu_lib/Basic_Blocks/DTC_Info
  Data Type Conversion : DataTypeConversion  OutDataTypeStr=uint8
  Data Type Conversion{1..2,8..9} (4 alike) : DataTypeConversion
  Data Type Conversion3 : DataTypeConversion  OutDataTypeStr=uint16
  Data Type Conversion4 : DataTypeConversion  OutDataTypeStr=uint8
  Data Type Conversion5 : DataTypeConversion  OutDataTypeStr=uint32
  Data Type Conversion6 : DataTypeConversion  OutDataTypeStr=uint16
  Divide{,1,7,11,16,20} (6 alike) : Product  Inputs=*/
  Equal10 : RelationalOperator  Operator=~=  OutDataTypeStr=boolean  RndMeth=Simplest
  Equal13 : RelationalOperator  Operator=~=  OutDataTypeStr=boolean  RndMeth=Simplest
  Equal8 : RelationalOperator  Operator===  OutDataTypeStr=boolean  RndMeth=Simplest
  Equal9 : RelationalOperator  Operator=~=  OutDataTypeStr=boolean  RndMeth=Simplest
  Logical Operator1 : Logic  Operator=NOT  AllPortsSameDT=off  OutDataTypeStr=boolean
  Logical Operator{25,28..31} (5 alike) : Logic  AllPortsSameDT=off  OutDataTypeStr=boolean
  Logical Operator27 : Logic  Operator=OR  AllPortsSameDT=off  OutDataTypeStr=boolean
  Logical Operator32 : Logic  Operator=OR  AllPortsSameDT=off  OutDataTypeStr=boolean
  Logical Operator33 : Logic  Operator=OR  AllPortsSameDT=off  OutDataTypeStr=boolean
  Relational Operator : RelationalOperator  Operator=>  OutDataTypeStr=boolean  RndMeth=Simplest
  Relational Operator1 : RelationalOperator  Operator=<=  OutDataTypeStr=boolean  RndMeth=Simplest
  Relational Operator12 : RelationalOperator  OutDataTypeStr=boolean  RndMeth=Simplest
  Relational Operator13 : RelationalOperator  Operator=<  OutDataTypeStr=boolean  RndMeth=Simplest
  Relational Operator2 : RelationalOperator  Operator=>  OutDataTypeStr=boolean  RndMeth=Simplest
  Relational Operator8 : RelationalOperator  Operator=<  OutDataTypeStr=boolean  RndMeth=Simplest
  Relational Operator9 : RelationalOperator  Operator=<=  OutDataTypeStr=boolean  RndMeth=Simplest
  Relay1 : Relay  OnSwitchValue=ONE_INT  OffSwitchValue=ZERO_INT
  SR_Latch2 : hcu_lib/Basic_Blocks/SR_Latch
  SR_Latch5 : hcu_lib/Basic_Blocks/SR_Latch
  Switch{1..3,6,8..9,13} (7 alike) : Switch  Criteria=u2 > Threshold
  Switch{4,7,11..12,15..16} (6 alike) : Switch  Criteria=u2 ~= 0
  Test Detection Criteria1 : hcu_lib/Basic_Blocks/Test Detection Criteria
  Unit Delay{1..3,5..6} (5 alike) : UnitDelay  SampleTime=-1  HasFrameUpgradeWarning=on
  VDDM_DrStSWDTC_raw32 : Outport
  Dr_SeatSta : Outport  Port=2
  wires:
  DTC_clear_request/1 -> [DTC_clear_request]
  VINP_DrStSW/1 -> [VINP_DrStSWGPIO_flg]
  task_time_s/1 -> [task_time_s]
  [VDDM_DrStSWCFS_flg] -> Switch11/2
  Constant42/1 -> Switch11/1
  Switch11/1 -> [Dr_SeatSta]
  Logical Operator27/1 -> Switch15/2
  Constant52/1 -> Switch16/1
  Equal8/1 -> Logical Operator27/1
  [VDDM_DrStSWPass_flg] -> Switch16/2
  Constant53/1 -> Switch16/3
  Constant45/1 -> Equal8/2
  Constant55/1 -> Switch15/3
  Switch15/1 -> [VDDM_DrStSWCFSRls_flg]
  Switch16/1 -> [VDDM_DrStSWDFSRls_flg]
  [DTC_clear_request] -> Logical Operator27/2
  Constant54/1 -> Switch15/1
  [VPMM_PowerSta_enum] -> Equal8/1
  Relay1/1 -> SR_Latch2/1
  [VDDM_DrStSWDet_flg] -> Logical Operator31/1
  Logical Operator29/1 -> DTC_Couter1/2
  [VDDM_DrStSWCFSRls_flg] -> SR_Latch5/2
  SR_Latch2/1 -> Logical Operator28/2
  SR_Latch5/1 -> Logical Operator30/1
  [VDDM_DrStSWDFSRls_flg] -> Logical Operator32/1
  Logical Operator32/1 -> SR_Latch2/2
  DTC_Couter1/2 -> Data Type Conversion4/1
  Logical Operator33/1 -> Logical Operator29/1
  Data Type Conversion4/1 -> [VDDM_DrStSWDTC_cnt]  "VDDM_DrStSWDTC_cnt"
  [VDDM_DrStSWDTC_cnt] -> Relay1/1
  Logical Operator31/1 -> DTC_Couter1/1
  [VDDM_DrStSWCFS_flg] -> Logical Operator32/2
  Constant57/1 -> Logical Operator30/2
  DTC_Couter1/1 -> SR_Latch5/1
  Constant59/1 -> Logical Operator31/2
  [VDDM_DrStSWCFSRls_flg] -> Logical Operator33/2
  Logical Operator28/1 -> [VDDM_DrStSWDFS_flg]
  [VDDM_DrStSWPass_flg] -> Logical Operator33/1
  Logical Operator30/1 -> [VDDM_DrStSWCFS_flg]
  Constant56/1 -> Logical Operator29/2
  Constant60/1 -> DTC_Couter1/3
  Constant58/1 -> Logical Operator28/1
  [Dr_SeatSta] -> Dr_SeatSta/1
  Unit Delay2/1 -> Relational Operator9/1
  Switch12/1 -> Unit Delay6/1
  Constant3/1 -> Add4/1
  Relational Operator9/1 -> Logical Operator25/2
  Data Type Conversion6/1 -> Relational Operator12/1, [VDDM_DrStSWPass_cnt]
  [VDDM_DrStSWChange_flg] -> Logical Operator25/1
  Switch3/1 -> Data Type Conversion3/1
  Constant2/1 -> Switch13/3
  [VDDM_DrStSWPass_cnt] -> Switch3/1, Relational Operator13/1
  Divide11/1 -> Relational Operator12/2
  Logical Operator1/1 -> Switch13/2
  Logical Operator25/1 -> Logical Operator1/1
  Data Type Conversion/1 -> Switch12/3
  Divide16/1 -> Data Type Conversion1/1
  Constant5/1 -> Divide11/1
  Data Type Conversion3/1 -> Add4/2
  Add4/1 -> Switch13/1
  Equal9/1 -> Switch12/2
  Relational Operator12/1 -> [VDDM_DrStSWPass_flg]
  Switch13/1 -> Switch12/1
  Divide7/1 -> Relational Operator9/2
  [VPMM_PwrStaSW_enum] -> Equal9/1
  Constant50/1 -> Equal9/2
  Unit Delay6/1 -> Data Type Conversion6/1
  Constant47/1 -> Data Type Conversion/1
  Constant49/1 -> Divide7/1
  Constant39/1 -> Divide16/1
  [VDDM_DrStSWHiLoCount_enum] -> Unit Delay2/1
  VPMM_PowerSta_enum/1 -> [VPMM_PowerSta_enum]
  VPMM_PwrStaSW_enum/1 -> [VPMM_PwrStaSW_enum]
  [VINP_DrStSWGPIO_flg] -> Switch11/3
  Relational Operator13/1 -> Switch3/2
  Data Type Conversion1/1 -> Switch3/3, Relational Operator13/2
  DTC_Info/1 -> VDDM_DrStSWDTC_raw32/1  "VDDM_DrStSWDTC_raw32"
  [VDDM_DrStSWPass_flg] -> DTC_Info/2
  [VDDM_DrStSWCFS_flg] -> DTC_Info/3
  [VDDM_DrStSWDet_flg] -> DTC_Info/1
  [task_time_s] -> Divide16/2
  [task_time_s] -> Divide7/2
  [task_time_s] -> Divide11/2
  Constant37/1 -> Equal13/2
  Constant12/1 -> Switch1/1
  Relational Operator1/1 -> [VDDM_DrStSWFailcntEN_flg]
  Switch9/1 -> Switch8/1
  Relational Operator/1 -> Equal10/2, Unit Delay3/1
  Unit Delay1/1 -> Data Type Conversion5/1
  Divide1/1 -> Relational Operator1/2
  [task_time_s] -> Divide/2
  Add3/1 -> Data Type Conversion8/1
  [VINP_DrStSWGPIO_flg] -> Relational Operator/1
  Constant29/1 -> Add2/2
  Unit Delay3/1 -> Equal10/1
  Data Type Conversion5/1 -> [VDDM_DrStSWHiLoCount_enum]
  Equal13/1 -> Switch7/2
  Add2/1 -> Switch6/3
  [task_time_s] -> Test Detection Criteria1/2
  Constant6/1 -> Divide20/1
  Constant13/1 -> Switch9/3
  Constant28/1 -> Relational Operator/2
  Relational Operator2/1 -> Switch1/2
  Divide/1 -> Relational Operator2/2
  [VDDM_DrStSWHiLoCount_enum] -> Add2/1
  [VDDM_DrStSWHiLoCount_enum] -> Relational Operator1/1
  Constant10/1 -> Test Detection Criteria1/4
  Data Type Conversion9/1 -> Relational Operator8/2, Switch2/3
  Data Type Conversion8/1 -> Switch9/1
  [VDDM_DrStSWfail_cnt] -> Switch1/3
  [task_time_s] -> Divide1/2
  Constant14/1 -> Divide1/1
  [VDDM_DrStSWChange_flg] -> Switch6/2
  Constant1/1 -> Switch7/3
  Constant4/1 -> Divide/1
  Test Detection Criteria1/1 -> [VDDM_DrStSWDet_flg]  "VDDM_DrStSWDet_flg"
  [VDDM_DrStSWfail_cnt] -> Relational Operator8/1, Switch2/1
  [task_time_s] -> Divide20/2
  [VDDM_DrStSWChange_flg] -> Switch8/2
  [VPMM_PwrStaSW_enum] -> Equal13/1
  [VDDM_DrStSWHiLoCount_enum] -> Relational Operator2/1
  Switch1/1 -> Switch8/3
  Switch8/1 -> Switch7/1
  Constant31/1 -> Switch6/1
  [VDDM_DrStSWHiLoCount_enum] -> Add3/1
  Switch7/1 -> Unit Delay5/1
  Switch2/1 -> Data Type Conversion2/1
  Switch6/1 -> Unit Delay1/1
  Data Type Conversion2/1 -> Add3/2
  [VDDM_DrStSWFailcntEN_flg] -> Switch9/2
  Relational Operator8/1 -> Switch2/2
  Equal10/1 -> [VDDM_DrStSWChange_flg]
  Constant11/1 -> Test Detection Criteria1/3
  Divide20/1 -> Data Type Conversion9/1
  [DTC_clear_request] -> DTC_Info/4
  [DTC_clear_request] -> Switch4/2
  Switch4/1 -> Test Detection Criteria1/1
  Unit Delay5/1 -> [VDDM_DrStSWfail_cnt], Switch4/3
  Constant7/1 -> Switch4/1

== system ddm/DDM/DDM/PMM/SW failure/FL Door switch failure ==
  note: Test Pass Criteria
  note: Test Detection Criteria
  note: Diagnostics and Fault Handling
  note: Release Condition During Detection
  note: Release Condition After Decision
  note: Fail Safe After Decision
  note: Fail Safe During Detection
  task_time_s : Inport
  VPMM_PowerSta_enum : Inport  Port=2
  VPMM_PwrStaSW_enum : Inport  Port=3
  VINP_FLAJARSW : Inport  Port=4
  DTC_clear_request : Inport  Port=5
  Add2 : Sum
  Add3 : Sum
  Add4 : Sum  AccumDataTypeStr=uint16
  Constant{1..2,12..13,31} (5 alike) : Constant  Value=ZERO_INT
  Constant14 : Constant  Value=KDDM_FLDoorSW_s
  Constant28 : Constant  Value=ZERO_FLOAT
  Constant29 : Constant  Value=ONE_INT
  Constant3 : Constant  Value=ONE_INT
  Constant37 : Constant  Value=ENUM_PWRSTASW_OFF
  Constant39 : Constant  Value=KDDM_FLDoorSWPassTO_s
  Constant4 : Constant  Value=KDDM_FLDoorSW_s
  Constant{42,47,52,54} (4 alike) : Constant  Value=TRUE
  Constant45 : Constant  Value=ENUM_POWERSTA_OFF
  Constant49 : Constant  Value=KDDM_FLDoorSW_s
  Constant5 : Constant  Value=KDDM_FLDoorSWDTC_cnt
  Constant50 : Constant  Value=ENUM_PWRSTASW_OFF
  Constant53 : Constant  Value=FALSE
  Constant55 : Constant  Value=FALSE
  Constant56 : Constant  Value=KDDM_FLDoorSWPassSW_flg
  Constant57 : Constant  Value=KDDM_FLDoorSWCFSSW_flg
  Constant58 : Constant  Value=KDDM_FLDoorSWDFSSW_flg
  Constant59 : Constant  Value=KDDM_FLDoorSWDetSW_flg
  Constant6 : Constant  Value=KDDM_FLDoorSWDetTO_s
  Constant60 : Constant  Value=KDDM_FLDoorSWDTC_cnt
  Constant7 : Constant  Value=KDDM_FLDoorSWPassTO_s
  Constant8 : Constant  Value=KDDM_FLDoorSWDetTO_s
  Constant9 : Constant  Value=FALSE
  DTC_Couter1 : hcu_lib/Basic_Blocks/DTC_Couter
  DTC_Info : hcu_lib/Basic_Blocks/DTC_Info
  Data Type Conversion : DataTypeConversion  OutDataTypeStr=uint8
  Data Type Conversion{1,7..9} (4 alike) : DataTypeConversion
  Data Type Conversion2 : DataTypeConversion  OutDataTypeStr=uint32
  Data Type Conversion3 : DataTypeConversion  OutDataTypeStr=uint16
  Data Type Conversion4 : DataTypeConversion  OutDataTypeStr=uint8
  Data Type Conversion5 : DataTypeConversion  OutDataTypeStr=uint32
  Data Type Conversion6 : DataTypeConversion  OutDataTypeStr=uint16
  Divide{,1,7,11,16,20} (6 alike) : Product  Inputs=*/
  Equal10 : RelationalOperator  Operator=~=  OutDataTypeStr=boolean  RndMeth=Simplest
  Equal13 : RelationalOperator  Operator=~=  OutDataTypeStr=boolean  RndMeth=Simplest
  Equal8 : RelationalOperator  Operator===  OutDataTypeStr=boolean  RndMeth=Simplest
  Equal9 : RelationalOperator  Operator=~=  OutDataTypeStr=boolean  RndMeth=Simplest
  Logical Operator1 : Logic  Operator=NOT  AllPortsSameDT=off  OutDataTypeStr=boolean
  Logical Operator{25,28..31} (5 alike) : Logic  AllPortsSameDT=off  OutDataTypeStr=boolean
  Logical Operator27 : Logic  Operator=OR  AllPortsSameDT=off  OutDataTypeStr=boolean
  Logical Operator32 : Logic  Operator=OR  AllPortsSameDT=off  OutDataTypeStr=boolean
  Logical Operator33 : Logic  Operator=OR  AllPortsSameDT=off  OutDataTypeStr=boolean
  Relational Operator : RelationalOperator  Operator=>  OutDataTypeStr=boolean  RndMeth=Simplest
  Relational Operator1 : RelationalOperator  Operator=<=  OutDataTypeStr=boolean  RndMeth=Simplest
  Relational Operator12 : RelationalOperator  OutDataTypeStr=boolean  RndMeth=Simplest
  Relational Operator13 : RelationalOperator  Operator=<  OutDataTypeStr=boolean  RndMeth=Simplest
  Relational Operator2 : RelationalOperator  Operator=>  OutDataTypeStr=boolean  RndMeth=Simplest
  Relational Operator8 : RelationalOperator  Operator=<  OutDataTypeStr=boolean  RndMeth=Simplest
  Relational Operator9 : RelationalOperator  Operator=<=  OutDataTypeStr=boolean  RndMeth=Simplest
  Relay1 : Relay  OnSwitchValue=ONE_INT  OffSwitchValue=ZERO_INT
  SR_Latch2 : hcu_lib/Basic_Blocks/SR_Latch
  SR_Latch5 : hcu_lib/Basic_Blocks/SR_Latch
  Switch{1..3,6,8..9,13} (7 alike) : Switch  Criteria=u2 > Threshold
  Switch{4,7,11..12,15..16} (6 alike) : Switch  Criteria=u2 ~= 0
  Test Detection Criteria1 : hcu_lib/Basic_Blocks/Test Detection Criteria
  Unit Delay{1..3,5..6} (5 alike) : UnitDelay  SampleTime=-1  HasFrameUpgradeWarning=on
  VDDM_FLDoorSWDTC_raw32 : Outport
  VCUFLDoorSta : Outport  Port=2
  wires:
  [VDDM_FLDoorSWHiLoCount_enum] -> Unit Delay2/1
  Constant39/1 -> Divide16/1
  Constant49/1 -> Divide7/1
  Constant47/1 -> Data Type Conversion/1
  Unit Delay6/1 -> Data Type Conversion6/1
  Constant50/1 -> Equal9/2
  [VPMM_PwrStaSW_enum] -> Equal9/1
  Divide7/1 -> Relational Operator9/2
  Switch13/1 -> Switch12/1
  Relational Operator12/1 -> [VDDM_FLDoorSWPass_flg]
  Equal9/1 -> Switch12/2
  Add4/1 -> Switch13/1
  Data Type Conversion3/1 -> Add4/2
  Constant7/1 -> Divide11/1
  Divide16/1 -> Data Type Conversion1/1
  Data Type Conversion/1 -> Switch12/3
  Logical Operator25/1 -> Logical Operator1/1
  Logical Operator1/1 -> Switch13/2
  Divide11/1 -> Relational Operator12/2
  [VDDM_FLDoorSWPass_cnt] -> Relational Operator13/1, Switch3/1
  Constant2/1 -> Switch13/3
  Switch3/1 -> Data Type Conversion3/1
  [VDDM_FLDoorSWChange_flg] -> Logical Operator25/1
  Data Type Conversion6/1 -> [VDDM_FLDoorSWPass_cnt], Relational Operator12/1
  Relational Operator9/1 -> Logical Operator25/2
  Constant3/1 -> Add4/1
  Switch12/1 -> Unit Delay6/1
  Unit Delay2/1 -> Relational Operator9/1
  Unit Delay5/1 -> Switch4/3, Data Type Conversion7/1
  Divide/1 -> Relational Operator2/2
  Switch8/1 -> Switch7/1
  [VDDM_FLDoorSWChange_flg] -> Switch8/2
  Constant6/1 -> Divide20/1
  Constant28/1 -> Relational Operator/2
  Relational Operator/1 -> Equal10/2, Unit Delay3/1
  Constant14/1 -> Divide1/1
  Constant13/1 -> Switch9/3
  [VDDM_FLDoorSWfail_cnt] -> Switch2/1, Relational Operator8/1
  [VDDM_FLDoorSWChange_flg] -> Switch6/2
  [VDDM_FLDoorSWHiLoCount_enum] -> Add3/1
  Constant8/1 -> Test Detection Criteria1/4
  Test Detection Criteria1/1 -> [VDDM_FLDoorSWDet_flg]  "VDDM_FLDoorSWDet_flg"
  Switch1/1 -> Switch8/3
  [VDDM_FLDoorSWFailcntEN_flg] -> Switch9/2
  [VDDM_FLDoorSWHiLoCount_enum] -> Relational Operator2/1
  Switch7/1 -> Unit Delay5/1
  [VPMM_PwrStaSW_enum] -> Equal13/1
  [VDDM_FLDoorSWfail_cnt] -> Switch1/3
  Equal13/1 -> Switch7/2
  Switch9/1 -> Switch8/1
  Constant4/1 -> Divide/1
  Add3/1 -> Data Type Conversion8/1
  Constant37/1 -> Equal13/2
  Constant12/1 -> Switch1/1
  Unit Delay1/1 -> Data Type Conversion5/1
  Switch6/1 -> Unit Delay1/1
  Constant29/1 -> Add2/2
  Constant1/1 -> Switch7/3
  Equal10/1 -> [VDDM_FLDoorSWChange_flg]
  Unit Delay3/1 -> Equal10/1
  Constant31/1 -> Switch6/1
  Relational Operator2/1 -> Switch1/2
  [VINP_FL_AJAR_SW] -> Relational Operator/1
  Add2/1 -> Switch6/3
  Divide20/1 -> Data Type Conversion9/1
  [VDDM_FLDoorSWHiLoCount_enum] -> Relational Operator1/1
  Relational Operator1/1 -> [VDDM_FLDoorSWFailcntEN_flg]
  Data Type Conversion5/1 -> [VDDM_FLDoorSWHiLoCount_enum]
  Divide1/1 -> Relational Operator1/2
  [VCUFLDoorSta] -> VCUFLDoorSta/1
  Constant58/1 -> Logical Operator28/1
  Constant60/1 -> DTC_Couter1/3
  Constant56/1 -> Logical Operator29/2
  Logical Operator30/1 -> [VDDM_FLDoorSWCFS_flg]
  [VDDM_FLDoorSWPass_flg] -> Logical Operator33/1
  Logical Operator28/1 -> [VDDM_FLDoorSWDFS_flg]
  [VDDM_FLDoorSWCFSRls_flg] -> Logical Operator33/2
  Constant59/1 -> Logical Operator31/2
  DTC_Couter1/1 -> SR_Latch5/1
  Constant57/1 -> Logical Operator30/2
  [VDDM_FLDoorSWCFS_flg] -> Logical Operator32/2
  Logical Operator31/1 -> DTC_Couter1/1
  [VDDM_FLDoorSWDTC_cnt] -> Relay1/1
  Data Type Conversion4/1 -> [VDDM_FLDoorSWDTC_cnt]  "VDDM_FLDoorSWDTC_cnt"
  Logical Operator33/1 -> Logical Operator29/1
  DTC_Couter1/2 -> Data Type Conversion4/1
  Logical Operator32/1 -> SR_Latch2/2
  [VDDM_FLDoorSWDFSRls_flg] -> Logical Operator32/1
  SR_Latch5/1 -> Logical Operator30/1
  SR_Latch2/1 -> Logical Operator28/2
  [VDDM_FLDoorSWCFSRls_flg] -> SR_Latch5/2
  Logical Operator29/1 -> DTC_Couter1/2
  [VDDM_FLDoorSWDet_flg] -> Logical Operator31/1
  Relay1/1 -> SR_Latch2/1
  [VPMM_PowerSta_enum] -> Equal8/1
  Constant54/1 -> Switch15/1
  [DTC_clear_request] -> Logical Operator27/2
  Switch16/1 -> [VDDM_FLDoorSWDFSRls_flg]
  Switch15/1 -> [VDDM_FLDoorSWCFSRls_flg]
  Constant55/1 -> Switch15/3
  Constant45/1 -> Equal8/2
  Constant53/1 -> Switch16/3
  [VDDM_FLDoorSWPass_flg] -> Switch16/2
  Equal8/1 -> Logical Operator27/1
  Constant52/1 -> Switch16/1
  Logical Operator27/1 -> Switch15/2
  Switch11/1 -> [VCUFLDoorSta]
  Constant42/1 -> Switch11/1
  [VDDM_FLDoorSWCFS_flg] -> Switch11/2
  task_time_s/1 -> [task_time_s]
  VINP_FLAJARSW/1 -> [VINP_FL_AJAR_SW]
  DTC_clear_request/1 -> [DTC_clear_request]
  VPMM_PwrStaSW_enum/1 -> [VPMM_PwrStaSW_enum]
  VPMM_PowerSta_enum/1 -> [VPMM_PowerSta_enum]
  [VINP_FL_AJAR_SW] -> Switch11/3
  Data Type Conversion9/1 -> Relational Operator8/2, Switch2/3
  Relational Operator8/1 -> Switch2/2
  Switch2/1 -> Data Type Conversion2/1
  Data Type Conversion2/1 -> Add3/2
  [VDDM_FLDoorSWHiLoCount_enum] -> Add2/1
  Data Type Conversion7/1 -> [VDDM_FLDoorSWfail_cnt]
  Relational Operator13/1 -> Switch3/2
  Data Type Conversion1/1 -> Relational Operator13/2, Switch3/3
  Data Type Conversion8/1 -> Switch9/1
  DTC_Info/1 -> VDDM_FLDoorSWDTC_raw32/1  "VDDM_FLDoorSWDTC_raw32"
  [VDDM_FLDoorSWPass_flg] -> DTC_Info/2
  [VDDM_FLDoorSWCFS_flg] -> DTC_Info/3
  [VDDM_FLDoorSWDet_flg] -> DTC_Info/1
  [task_time_s] -> Divide1/2
  [task_time_s] -> Divide20/2
  [task_time_s] -> Divide/2
  [task_time_s] -> Test Detection Criteria1/2
  [task_time_s] -> Divide16/2
  [task_time_s] -> Divide7/2
  [task_time_s] -> Divide11/2
  Constant5/1 -> Test Detection Criteria1/3
  [DTC_clear_request] -> DTC_Info/4
  [DTC_clear_request] -> Switch4/2
  Switch4/1 -> Test Detection Criteria1/1
  Constant9/1 -> Switch4/1
